simulink model "modeloFdeT"  (R2024b)
settings: Solver=VariableStepAuto  StartTime=0.0  StopTime=10.0  RelTol=1e-3
settings Model: Creator=estel  LastModifiedBy=estel

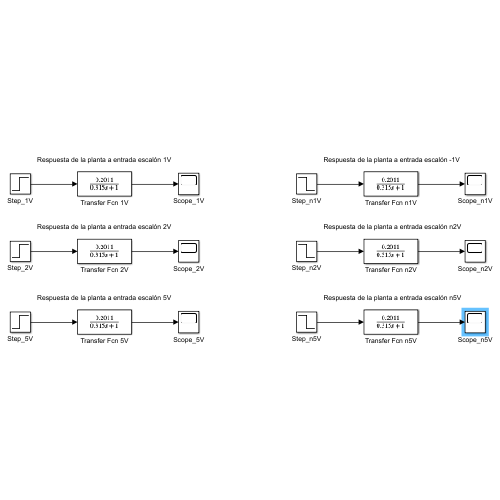
[thumbnail: Simulink's stored preview of the top-level diagram]
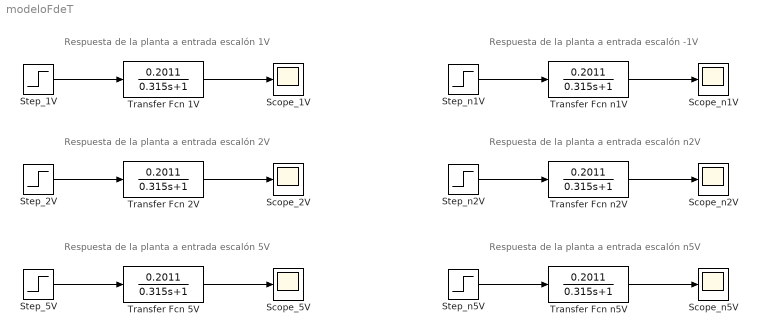
== system modeloFdeT ==
  note: Respuesta de la planta a entrada escalón 1V
  note: Respuesta de la planta a entrada escalón 2V
  note: Respuesta de la planta a entrada escalón 5V
  note: Respuesta de la planta a entrada escalón n5V
  note: Respuesta de la planta a entrada escalón n2V
  note: Respuesta de la planta a entrada escalón -1V
  Scope_1V : Scope
  Scope_2V : Scope
  Scope_5V : Scope
  Scope_n1V : Scope
  Scope_n2V : Scope
  Scope_n5V : Scope
  Step_1V : Step  SampleTime=0
  Step_2V : Step  After=2  SampleTime=0
  Step_5V : Step  After=5  SampleTime=0
  Step_n1V : Step  After=-1  SampleTime=0
  Step_n2V : Step  After=-2  SampleTime=0
  Step_n5V : Step  After=-5  SampleTime=0
  Transfer Fcn 1V : TransferFcn  Numerator=0.2011  Denominator=[0.315 1]
  Transfer Fcn 2V : TransferFcn  Numerator=0.2011  Denominator=[0.315 1]
  Transfer Fcn 5V : TransferFcn  Numerator=0.2011  Denominator=[0.315 1]
  Transfer Fcn n1V : TransferFcn  Numerator=0.2011  Denominator=[0.315 1]
  Transfer Fcn n2V : TransferFcn  Numerator=0.2011  Denominator=[0.315 1]
  Transfer Fcn n5V : TransferFcn  Numerator=0.2011  Denominator=[0.315 1]
  wires:
  Step_1V/1 -> Transfer Fcn 1V/1
  Transfer Fcn 1V/1 -> Scope_1V/1
  Step_n5V/1 -> Transfer Fcn n5V/1
  Transfer Fcn n5V/1 -> Scope_n5V/1
  Step_n2V/1 -> Transfer Fcn n2V/1
  Transfer Fcn n2V/1 -> Scope_n2V/1
  Transfer Fcn n1V/1 -> Scope_n1V/1
  Step_n1V/1 -> Transfer Fcn n1V/1
  Step_2V/1 -> Transfer Fcn 2V/1
  Transfer Fcn 2V/1 -> Scope_2V/1
  Step_5V/1 -> Transfer Fcn 5V/1
  Transfer Fcn 5V/1 -> Scope_5V/1
